simulink model "ramp_ball_animation"  (R2015a)
settings: Solver=ode45  StartTime=0.0  StopTime=inf  RelTol=1e-3
undefined symbols (not defined in the file or in its folder): drawRamp
libraries: simulink x1
settings Model: Creator=ecestudent  LastModifiedBy=ecestudent

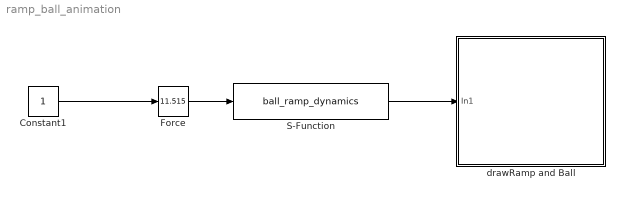
== system ramp_ball_animation ==
  Constant1 : Constant
  Force : simulink/Math Operations/Slider Gain  low=0  gain=11.515  high=20
  S-Function : S-Function  FunctionName=ball_ramp_dynamics  Parameters=ramp_ball_params
  drawRamp and Ball : Subsystem
      mask Display: image(imread('tv.jpg'))
  wires:
  Constant1/1 -> Force/1
  S-Function/1 -> drawRamp and Ball/1(In1)
  Force/1 -> S-Function/1

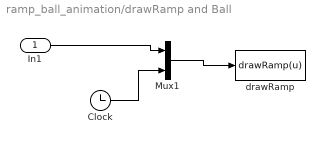
== system ramp_ball_animation/drawRamp and Ball ==
  In1 : Inport
  Clock : Clock
  Mux1 : Mux  Inputs=2
  drawRamp : MATLABFcn  MATLABFcn=drawRamp(u)  OutputDimensions=0
  wires:
  In1/1 -> Mux1/1
  Clock/1 -> Mux1/2
  Mux1/1 -> drawRamp/1
